simulink model "model"  (R2019a)
settings: Solver=FixedStepDiscrete  StartTime=0.0  StopTime=8  FixedStep=1/30  RelTol=1e-3  EnableMultiTasking=on
values from neighbouring files (symbols this model uses):
  A0 = 914.02    [parameter.mat]
  A1 = 12.9    [parameter.mat]
  A2 = 2028.24    [parameter.mat]
  b = 1.14    [parameter.mat]
  bpitch = 4000    [parameter.mat]
  broll = 4000    [parameter.mat]
  c = 1.14    [parameter.mat]
  C1 = 1    [parameter.mat]
  C2 = 0.34    [parameter.mat]
  C3 = 0.57    [parameter.mat]
  C4 = 0.32    [parameter.mat]
  CF = 18.7    [parameter.mat]
  f = 1.215    [parameter.mat]
  Fzt = 810    [parameter.mat]
  hs = 0.55    [parameter.mat]
  ip = 50    [parameter.mat]
  ir = 425    [parameter.mat]
  iw = 1.1    [parameter.mat]
  iz = 3136    [parameter.mat]
  Ka = 0.05    [parameter.mat]
  kpitch = 170000    [parameter.mat]
  kroll = 90000    [parameter.mat]
  m = 750    [parameter.mat]
  miudot = 0.85    [parameter.mat]
  ms = 650    [parameter.mat]
  r = 1.205    [parameter.mat]
  rw = 0.237    [parameter.mat]
  Tp = 24    [parameter.mat]
  Tw = 6    [parameter.mat]
  w = 2.28    [parameter.mat]
undefined symbols (not defined in the file or in its folder): DiscIntNeverNeededParam, Rec, SDTV, sigbuilder_block
libraries: dspmtrx3 x3, visionconversions x2, visiontextngfix x2, visiontransforms x2, fuzblock x1, dspvision x1, visionfilter x1, visionsinks x1, visionstatistics x1
(part 2 of 3)

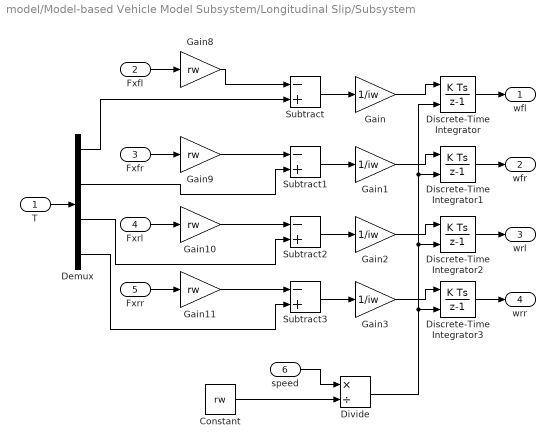
== system model/Model-based Vehicle Model Subsystem/Longitudinal Slip/Subsystem ==
  T : Inport
  Fxfl : Inport  Port=2
  Fxfr : Inport  Port=3
  Fxrl : Inport  Port=4
  Fxrr : Inport  Port=5
  speed : Inport  Port=6
  Constant : Constant  Value=rw
  Demux : Demux
  Discrete-Time Integrator{,1..3} (4 alike) : DiscreteIntegrator  InitialConditionSource=external  InitialCondition=22.222/rw  SampleTime=-1  LimitOutput=on  LowerSaturationLimit=0  ICPrevOutput=DiscIntNeverNeededParam  ICPrevScaledInput=DiscIntNeverNeededParam
  Divide : Product  Inputs=*/
  Gain{,1..3} (4 alike) : Gain  Gain=1/iw
  Gain{8..11} (4 alike) : Gain  Gain=rw
  Subtract{,1..3} (4 alike) : Sum  Inputs=-+
  wfl : Outport
  wfr : Outport  Port=2
  wrl : Outport  Port=3
  wrr : Outport  Port=4
  wires:
  Fxfl/1 -> Gain8/1
  Fxfr/1 -> Gain9/1
  Fxrl/1 -> Gain10/1
  Fxrr/1 -> Gain11/1
  Subtract/1 -> Gain/1
  Subtract1/1 -> Gain1/1
  Subtract2/1 -> Gain2/1
  Subtract3/1 -> Gain3/1
  Gain8/1 -> Subtract/1
  Gain9/1 -> Subtract1/1
  T/1 -> Demux/1
  Demux/1 -> Subtract/2
  Demux/2 -> Subtract1/2
  Demux/3 -> Subtract2/2
  Demux/4 -> Subtract3/2
  Gain/1 -> Discrete-Time Integrator/1
  Gain1/1 -> Discrete-Time Integrator1/1
  Gain2/1 -> Discrete-Time Integrator2/1
  Gain3/1 -> Discrete-Time Integrator3/1
  Discrete-Time Integrator/1 -> wfl/1
  Discrete-Time Integrator1/1 -> wfr/1
  Discrete-Time Integrator2/1 -> wrl/1
  Discrete-Time Integrator3/1 -> wrr/1
  Gain10/1 -> Subtract2/1
  Gain11/1 -> Subtract3/1
  speed/1 -> Divide/1
  Constant/1 -> Divide/2
  Divide/1 -> Discrete-Time Integrator2/2, Discrete-Time Integrator1/2, Discrete-Time Integrator/2, Discrete-Time Integrator3/2

== system model/Model-based Vehicle Model Subsystem/Longitudinal Slip/fl ==
  ax : Inport
  ay : Inport  Port=2
  Alpha_fl : Inport  Port=3
  yaw_rate : Inport  Port=4
  wfl : Inport  Port=5
  speed : Inport  Port=6
  Add1 : Sum
  Discrete-Time Integrator : DiscreteIntegrator  InitialConditionSource=external  InitialCondition=22.222  SampleTime=-1  LimitOutput=on  LowerSaturationLimit=0  ICPrevOutput=DiscIntNeverNeededParam  ICPrevScaledInput=DiscIntNeverNeededParam
  Discrete-Time Integrator1 : DiscreteIntegrator  SampleTime=-1  ICPrevOutput=DiscIntNeverNeededParam  ICPrevScaledInput=DiscIntNeverNeededParam
  Divide : Product  Inputs=*/
  Gain1 : Gain  Gain=b
  Gain2 : Gain  Gain=rw
  Math Function : Math  Operator=square  SaturateOnIntegerOverflow=on
  Math Function1 : Math  Operator=square  SaturateOnIntegerOverflow=on
  Math Function2 : Math  Operator=sqrt  SaturateOnIntegerOverflow=on
  Product1 : Product  RndMeth=Zero
  Saturation : Saturate  UpperLimit=1  LowerLimit=-1
  Subtract : Sum
  Subtract1 : Sum  Inputs=+-
  Trigonometric Function : Trigonometry  Operator=cos
  Sfl : Outport
  wires:
  ax/1 -> Discrete-Time Integrator/1
  wfl/1 -> Gain2/1
  ay/1 -> Discrete-Time Integrator1/1
  Math Function/1 -> Add1/1
  Add1/1 -> Math Function2/1
  Math Function2/1 -> Product1/1
  yaw_rate/1 -> Gain1/1
  Gain1/1 -> Subtract/2
  Subtract/1 -> Math Function1/1
  Math Function1/1 -> Add1/2
  Alpha_fl/1 -> Trigonometric Function/1
  Trigonometric Function/1 -> Product1/2
  Divide/1 -> Saturation/1
  Subtract1/1 -> Divide/1
  Product1/1 -> Divide/2, Subtract1/2
  Saturation/1 -> Sfl/1
  Gain2/1 -> Subtract1/1
  Discrete-Time Integrator/1 -> Math Function/1
  Discrete-Time Integrator1/1 -> Subtract/1
  speed/1 -> Discrete-Time Integrator/2

== system model/Model-based Vehicle Model Subsystem/Longitudinal Slip/fr ==
  ax : Inport
  vy : Inport  Port=2
  Alpha_fr : Inport  Port=3
  yaw_rate : Inport  Port=4
  wfr : Inport  Port=5
  speed : Inport  Port=6
  Add1 : Sum
  Discrete-Time Integrator : DiscreteIntegrator  InitialConditionSource=external  InitialCondition=22.222  SampleTime=-1  LimitOutput=on  LowerSaturationLimit=0  ICPrevOutput=DiscIntNeverNeededParam  ICPrevScaledInput=DiscIntNeverNeededParam
  Discrete-Time Integrator1 : DiscreteIntegrator  SampleTime=-1  ICPrevOutput=DiscIntNeverNeededParam  ICPrevScaledInput=DiscIntNeverNeededParam
  Divide : Product  Inputs=*/
  Gain1 : Gain  Gain=b
  Gain2 : Gain  Gain=rw
  Math Function : Math  Operator=square  SaturateOnIntegerOverflow=on
  Math Function1 : Math  Operator=square  SaturateOnIntegerOverflow=on
  Math Function2 : Math  Operator=sqrt  SaturateOnIntegerOverflow=on
  Product1 : Product  RndMeth=Zero
  Saturation : Saturate  UpperLimit=1  LowerLimit=-1
  Subtract : Sum
  Subtract1 : Sum  Inputs=+-
  Trigonometric Function : Trigonometry  Operator=cos
  Sfr : Outport
  wires:
  wfr/1 -> Gain2/1
  vy/1 -> Discrete-Time Integrator1/1
  Math Function/1 -> Add1/1
  Add1/1 -> Math Function2/1
  Math Function2/1 -> Product1/1
  yaw_rate/1 -> Gain1/1
  Gain1/1 -> Subtract/2
  Subtract/1 -> Math Function1/1
  Math Function1/1 -> Add1/2
  Alpha_fr/1 -> Trigonometric Function/1
  Trigonometric Function/1 -> Product1/2
  ax/1 -> Discrete-Time Integrator/1
  Subtract1/1 -> Divide/1
  Divide/1 -> Saturation/1
  Product1/1 -> Divide/2, Subtract1/2
  Saturation/1 -> Sfr/1
  Gain2/1 -> Subtract1/1
  Discrete-Time Integrator/1 -> Math Function/1
  Discrete-Time Integrator1/1 -> Subtract/1
  speed/1 -> Discrete-Time Integrator/2

== system model/Model-based Vehicle Model Subsystem/Longitudinal Slip/rl ==
  vx : Inport
  vy : Inport  Port=2
  Alpha_rl : Inport  Port=3
  yaw_rate : Inport  Port=4
  wrl : Inport  Port=5
  speed : Inport  Port=6
  Add1 : Sum
  Discrete-Time Integrator : DiscreteIntegrator  InitialConditionSource=external  InitialCondition=22.222  SampleTime=-1  LimitOutput=on  LowerSaturationLimit=0  ICPrevOutput=DiscIntNeverNeededParam  ICPrevScaledInput=DiscIntNeverNeededParam
  Discrete-Time Integrator1 : DiscreteIntegrator  SampleTime=-1  ICPrevOutput=DiscIntNeverNeededParam  ICPrevScaledInput=DiscIntNeverNeededParam
  Divide : Product  Inputs=*/
  Gain1 : Gain  Gain=c
  Gain2 : Gain  Gain=rw
  Math Function : Math  Operator=square  SaturateOnIntegerOverflow=on
  Math Function1 : Math  Operator=square  SaturateOnIntegerOverflow=on
  Math Function2 : Math  Operator=sqrt  SaturateOnIntegerOverflow=on
  Product1 : Product  RndMeth=Zero
  Saturation : Saturate  UpperLimit=1  LowerLimit=-1
  Subtract : Sum
  Subtract1 : Sum  Inputs=+-
  Trigonometric Function : Trigonometry  Operator=cos
  Srl : Outport
  wires:
  wrl/1 -> Gain2/1
  vy/1 -> Discrete-Time Integrator1/1
  Math Function/1 -> Add1/1
  Add1/1 -> Math Function2/1
  Math Function2/1 -> Product1/1
  yaw_rate/1 -> Gain1/1
  Gain1/1 -> Subtract/2
  Subtract/1 -> Math Function1/1
  Math Function1/1 -> Add1/2
  Alpha_rl/1 -> Trigonometric Function/1
  Trigonometric Function/1 -> Product1/2
  vx/1 -> Discrete-Time Integrator/1
  Subtract1/1 -> Divide/1
  Divide/1 -> Saturation/1
  Product1/1 -> Divide/2, Subtract1/2
  Saturation/1 -> Srl/1
  Gain2/1 -> Subtract1/1
  Discrete-Time Integrator/1 -> Math Function/1
  Discrete-Time Integrator1/1 -> Subtract/1
  speed/1 -> Discrete-Time Integrator/2

== system model/Model-based Vehicle Model Subsystem/Longitudinal Slip/rr ==
  vx : Inport
  vy : Inport  Port=2
  Alpha_rr : Inport  Port=3
  yaw_rate : Inport  Port=4
  wrr : Inport  Port=5
  speed : Inport  Port=6
  Add1 : Sum
  Discrete-Time Integrator : DiscreteIntegrator  InitialConditionSource=external  InitialCondition=22.222  SampleTime=-1  LimitOutput=on  LowerSaturationLimit=0  ICPrevOutput=DiscIntNeverNeededParam  ICPrevScaledInput=DiscIntNeverNeededParam
  Discrete-Time Integrator1 : DiscreteIntegrator  SampleTime=-1  ICPrevOutput=DiscIntNeverNeededParam  ICPrevScaledInput=DiscIntNeverNeededParam
  Divide : Product  Inputs=*/
  Gain1 : Gain  Gain=c
  Gain2 : Gain  Gain=rw
  Math Function : Math  Operator=square  SaturateOnIntegerOverflow=on
  Math Function1 : Math  Operator=square  SaturateOnIntegerOverflow=on
  Math Function2 : Math  Operator=sqrt  SaturateOnIntegerOverflow=on
  Product1 : Product  RndMeth=Zero
  Saturation : Saturate  UpperLimit=1  LowerLimit=-1
  Subtract : Sum
  Subtract1 : Sum  Inputs=+-
  Trigonometric Function : Trigonometry  Operator=cos
  Srr : Outport
  wires:
  wrr/1 -> Gain2/1
  vy/1 -> Discrete-Time Integrator1/1
  Math Function/1 -> Add1/1
  Add1/1 -> Math Function2/1
  Math Function2/1 -> Product1/1
  yaw_rate/1 -> Gain1/1
  Gain1/1 -> Subtract/2
  Subtract/1 -> Math Function1/1
  Math Function1/1 -> Add1/2
  Alpha_rr/1 -> Trigonometric Function/1
  Trigonometric Function/1 -> Product1/2
  vx/1 -> Discrete-Time Integrator/1
  Subtract1/1 -> Divide/1
  Divide/1 -> Saturation/1
  Product1/1 -> Divide/2, Subtract1/2
  Saturation/1 -> Srr/1
  Gain2/1 -> Subtract1/1
  Discrete-Time Integrator/1 -> Math Function/1
  Discrete-Time Integrator1/1 -> Subtract/1
  speed/1 -> Discrete-Time Integrator/2

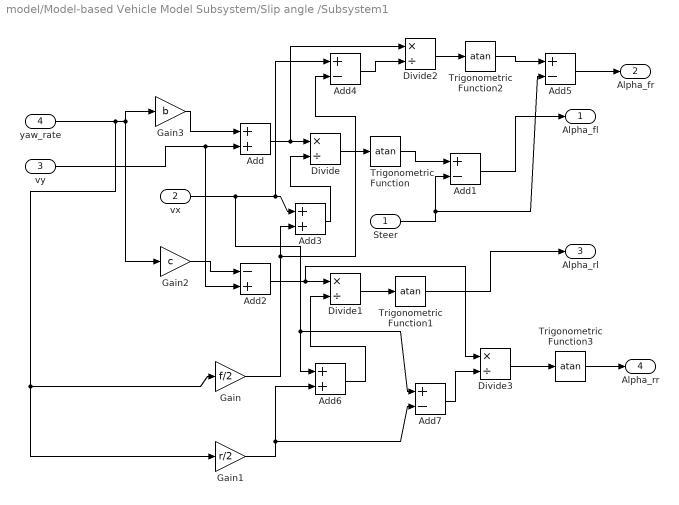
== system model/Model-based Vehicle Model Subsystem/Slip angle /Subsystem1 ==
  Steer : Inport
  vx : Inport  Port=2
  vy : Inport  Port=3
  yaw_rate : Inport  Port=4
  Add : Sum
  Add{1,4..5,7} (4 alike) : Sum  Inputs=+-
  Add2 : Sum  Inputs=-+
  Add3 : Sum
  Add6 : Sum
  Divide{,1..3} (4 alike) : Product  Inputs=*/
  Gain : Gain  Gain=f/2
  Gain1 : Gain  Gain=r/2
  Gain2 : Gain  Gain=c
  Gain3 : Gain  Gain=b
  Trigonometric Function{,1..3} (4 alike) : Trigonometry  Operator=atan
  Alpha_fl : Outport
  Alpha_fr : Outport  Port=2
  Alpha_rl : Outport  Port=3
  Alpha_rr : Outport  Port=4
  wires:
  yaw_rate/1 -> Gain1/1, Gain/1, Gain3/1, Gain2/1
  Gain3/1 -> Add/1
  vy/1 -> Add/2, Add2/2
  Add/1 -> Divide/1, Divide2/1
  Divide/1 -> Trigonometric Function/1
  Trigonometric Function/1 -> Add1/1
  Steer/1 -> Add1/2, Add5/2
  Add1/1 -> Alpha_fl/1
  Gain2/1 -> Add2/1
  Add2/1 -> Divide1/1, Divide3/1
  Divide1/1 -> Trigonometric Function1/1
  Trigonometric Function1/1 -> Alpha_rl/1
  vx/1 -> Add3/1, Add4/1, Add6/1, Add7/1
  Gain/1 -> Add3/2, Add4/2
  Add3/1 -> Divide/2
  Add4/1 -> Divide2/2
  Divide2/1 -> Trigonometric Function2/1
  Trigonometric Function2/1 -> Add5/1
  Add5/1 -> Alpha_fr/1
  Gain1/1 -> Add6/2, Add7/2
  Add6/1 -> Divide1/2
  Add7/1 -> Divide3/2
  Divide3/1 -> Trigonometric Function3/1
  Trigonometric Function3/1 -> Alpha_rr/1

== system model/Model-based Vehicle Model Subsystem/Slip angle /yaw effect motion ==
  ax : Inport
  ay : Inport  Port=2
  yaw_rate : Inport  Port=3
  speed : Inport  Port=4
  Add : Sum  Inputs=-+
  Add1 : Sum
  Discrete-Time Integrator : DiscreteIntegrator  SampleTime=-1  ICPrevOutput=DiscIntNeverNeededParam  ICPrevScaledInput=DiscIntNeverNeededParam
  Discrete-Time Integrator1 : DiscreteIntegrator  InitialConditionSource=external  InitialCondition=22.222  SampleTime=-1  LimitOutput=on  LowerSaturationLimit=0  ICPrevOutput=DiscIntNeverNeededParam  ICPrevScaledInput=DiscIntNeverNeededParam
  Product : Product  RndMeth=Zero
  Product1 : Product  RndMeth=Zero
  vx : Outport
  vy : Outport  Port=2
  wires:
  ay/1 -> Add/2
  Product/1 -> Add/1
  yaw_rate/1 -> Product/1, Product1/1
  Add/1 -> Discrete-Time Integrator/1
  Discrete-Time Integrator/1 -> vy/1, Product1/2
  ax/1 -> Add1/2
  Product1/1 -> Add1/1
  Add1/1 -> Discrete-Time Integrator1/1
  Discrete-Time Integrator1/1 -> vx/1, Product/2
  speed/1 -> Discrete-Time Integrator1/2

== system model/Model-based Vehicle Model Subsystem/Tire Model/Subsystem ==
  sfl : Inport
  Fzfl : Inport  Port=2
  Alpha_fl : Inport  Port=3
  Subsystem : Subsystem
  Subsystem1 : Subsystem
  Subsystem2 : Subsystem
  Subsystem3 : Subsystem
  Subsystem4 : Subsystem
  Subsystem5 : Subsystem
  Subsystem6 : Subsystem
  Subsystem7 : Subsystem
  Subsystem8 : Subsystem
  Unit Delay : UnitDelay  SampleTime=1/30  HasFrameUpgradeWarning=on
  Fxfl : Outport
  Fyfl : Outport  Port=2
  wires:
  Fzfl/1 -> Subsystem1/3(Fz), Subsystem2/1(Fz), Subsystem3/1(Fz), Subsystem/1(Fz), Subsystem4/2(Fz), Subsystem7/2(Fz)
  Subsystem/1(apdot) -> Subsystem1/1(apdot), Subsystem2/2(apdot), Subsystem3/2(apdot)
  Subsystem1/1(ap) -> Subsystem4/1(ap)
  Subsystem2/1(Kc) -> Subsystem4/4(Kc), Subsystem6/1(Kc)
  Subsystem3/1(Ks) -> Subsystem4/3(Ks), Subsystem6/2(Ks), Subsystem7/4(Ks), Subsystem8/3(Ks)
  sfl/1 -> Subsystem4/5(s), Subsystem6/3(s), Subsystem7/3(s)
  Alpha_fl/1 -> Subsystem4/6(Alpha), Subsystem6/4(Alpha), Subsystem7/6(Alpha), Subsystem8/5(Alpha)
  Subsystem4/1(gama) -> Subsystem5/1(gama)
  Subsystem7/1(Fx) -> Unit Delay/1, Fxfl/1
  Subsystem5/1(f(gama)) -> Subsystem7/5(f(gama)), Subsystem8/4(f(gama))
  Subsystem6/1(K'c) -> Subsystem7/1(K'c)
  Subsystem8/1(Fy) -> Fyfl/1
  Unit Delay/1 -> Subsystem1/2(Fx)
  Subsystem7/2(out1) -> Subsystem8/1(in1)
  Subsystem7/3(out2) -> Subsystem8/2(in2)

== system model/Model-based Vehicle Model Subsystem/Tire Model/Subsystem1 ==
  sfr : Inport
  Fzfr : Inport  Port=2
  Alpha_fr : Inport  Port=3
  Subsystem : Subsystem
  Subsystem1 : Subsystem
  Subsystem2 : Subsystem
  Subsystem3 : Subsystem
  Subsystem4 : Subsystem
  Subsystem5 : Subsystem
  Subsystem6 : Subsystem
  Subsystem7 : Subsystem
  Subsystem8 : Subsystem
  Unit Delay : UnitDelay  SampleTime=1/30  HasFrameUpgradeWarning=on
  Fxfr : Outport
  Fyfr : Outport  Port=2
  wires:
  Fzfr/1 -> Subsystem1/3(Fz), Subsystem2/1(Fz), Subsystem3/1(Fz), Subsystem/1(Fz), Subsystem4/2(Fz), Subsystem7/2(Fz)
  Subsystem/1(apdot) -> Subsystem1/1(apdot), Subsystem2/2(apdot), Subsystem3/2(apdot)
  Subsystem1/1(ap) -> Subsystem4/1(ap)
  Subsystem2/1(Kc) -> Subsystem4/4(Kc), Subsystem6/1(Kc)
  Subsystem3/1(Ks) -> Subsystem4/3(Ks), Subsystem6/2(Ks), Subsystem7/4(Ks), Subsystem8/3(Ks)
  sfr/1 -> Subsystem4/5(s), Subsystem6/3(s), Subsystem7/3(s)
  Alpha_fr/1 -> Subsystem4/6(Alpha), Subsystem6/4(Alpha), Subsystem7/6(Alpha), Subsystem8/5(Alpha)
  Subsystem4/1(gama) -> Subsystem5/1(gama)
  Subsystem7/1(Fx) -> Unit Delay/1, Fxfr/1
  Subsystem5/1(f(gama)) -> Subsystem7/5(f(gama)), Subsystem8/4(f(gama))
  Subsystem6/1(K'c) -> Subsystem7/1(K'c)
  Subsystem8/1(Fy) -> Fyfr/1
  Unit Delay/1 -> Subsystem1/2(Fx)
  Subsystem7/2(out1) -> Subsystem8/1(in1)
  Subsystem7/3(out2) -> Subsystem8/2(in2)

== system model/Model-based Vehicle Model Subsystem/Tire Model/Subsystem2 ==
  srl : Inport
  Fzrl : Inport  Port=2
  Alpha_rl : Inport  Port=3
  Subsystem : Subsystem
  Subsystem1 : Subsystem
  Subsystem2 : Subsystem
  Subsystem3 : Subsystem
  Subsystem4 : Subsystem
  Subsystem5 : Subsystem
  Subsystem6 : Subsystem
  Subsystem7 : Subsystem
  Subsystem8 : Subsystem
  Unit Delay : UnitDelay  SampleTime=1/30  HasFrameUpgradeWarning=on
  Fxrl : Outport
  Fyrl : Outport  Port=2
  wires:
  Fzrl/1 -> Subsystem1/3(Fz), Subsystem2/1(Fz), Subsystem3/1(Fz), Subsystem/1(Fz), Subsystem4/2(Fz), Subsystem7/2(Fz)
  Subsystem/1(apdot) -> Subsystem1/1(apdot), Subsystem2/2(apdot), Subsystem3/2(apdot)
  Subsystem1/1(ap) -> Subsystem4/1(ap)
  Subsystem2/1(Kc) -> Subsystem4/4(Kc), Subsystem6/1(Kc)
  Subsystem3/1(Ks) -> Subsystem4/3(Ks), Subsystem6/2(Ks), Subsystem7/4(Ks), Subsystem8/3(Ks)
  srl/1 -> Subsystem4/5(s), Subsystem6/3(s), Subsystem7/3(s)
  Alpha_rl/1 -> Subsystem4/6(Alpha), Subsystem6/4(Alpha), Subsystem7/6(Alpha), Subsystem8/5(Alpha)
  Subsystem4/1(gama) -> Subsystem5/1(gama)
  Subsystem7/1(Fx) -> Fxrl/1, Unit Delay/1
  Subsystem5/1(f(gama)) -> Subsystem7/5(f(gama)), Subsystem8/4(f(gama))
  Subsystem6/1(K'c) -> Subsystem7/1(K'c)
  Subsystem8/1(Fy) -> Fyrl/1
  Unit Delay/1 -> Subsystem1/2(Fx)
  Subsystem7/2(out1) -> Subsystem8/1(in1)
  Subsystem7/3(out2) -> Subsystem8/2(in2)

== system model/Model-based Vehicle Model Subsystem/Tire Model/Subsystem3 ==
  srr : Inport
  Fzrr : Inport  Port=2
  Alpha_rr : Inport  Port=3
  Subsystem : Subsystem
  Subsystem1 : Subsystem
  Subsystem2 : Subsystem
  Subsystem3 : Subsystem
  Subsystem4 : Subsystem
  Subsystem5 : Subsystem
  Subsystem6 : Subsystem
  Subsystem7 : Subsystem
  Subsystem8 : Subsystem
  Unit Delay : UnitDelay  SampleTime=1/30  HasFrameUpgradeWarning=on
  Fxrr : Outport
  Fyrr : Outport  Port=2
  wires:
  Fzrr/1 -> Subsystem1/3(Fz), Subsystem2/1(Fz), Subsystem3/1(Fz), Subsystem/1(Fz), Subsystem4/2(Fz), Subsystem7/2(Fz)
  Subsystem/1(apdot) -> Subsystem1/1(apdot), Subsystem2/2(apdot), Subsystem3/2(apdot)
  Subsystem1/1(ap) -> Subsystem4/1(ap)
  Subsystem2/1(Kc) -> Subsystem4/4(Kc), Subsystem6/1(Kc)
  Subsystem3/1(Ks) -> Subsystem4/3(Ks), Subsystem6/2(Ks), Subsystem7/4(Ks), Subsystem8/3(Ks)
  srr/1 -> Subsystem4/5(s), Subsystem6/3(s), Subsystem7/3(s)
  Alpha_rr/1 -> Subsystem4/6(Alpha), Subsystem6/4(Alpha), Subsystem7/6(Alpha), Subsystem8/5(Alpha)
  Subsystem4/1(gama) -> Subsystem5/1(gama)
  Subsystem7/1(Fx) -> Fxrr/1, Unit Delay/1
  Subsystem5/1(f(gama)) -> Subsystem7/5(f(gama)), Subsystem8/4(f(gama))
  Subsystem6/1(K'c) -> Subsystem7/1(K'c)
  Subsystem8/1(Fy) -> Fyrr/1
  Unit Delay/1 -> Subsystem1/2(Fx)
  Subsystem7/2(out1) -> Subsystem8/1(in1)
  Subsystem7/3(out2) -> Subsystem8/2(in2)

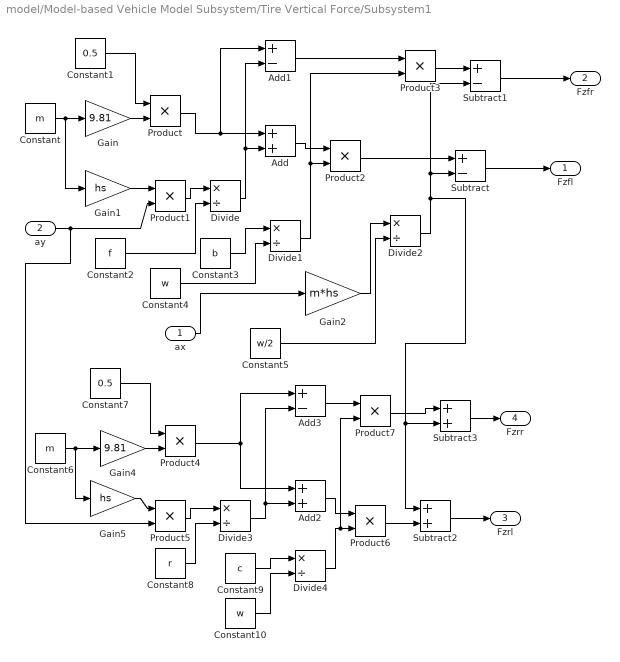
== system model/Model-based Vehicle Model Subsystem/Tire Vertical Force/Subsystem1 ==
  ax : Inport
  ay : Inport  Port=2
  Add : Sum
  Add1 : Sum  Inputs=+-
  Add2 : Sum
  Add3 : Sum  Inputs=+-
  Constant : Constant  Value=m
  Constant1 : Constant  Value=0.5
  Constant10 : Constant  Value=w
  Constant2 : Constant  Value=f
  Constant3 : Constant  Value=b
  Constant4 : Constant  Value=w
  Constant5 : Constant  Value=w/2
  Constant6 : Constant  Value=m
  Constant7 : Constant  Value=0.5
  Constant8 : Constant  Value=r
  Constant9 : Constant  Value=c
  Divide{,1..4} (5 alike) : Product  Inputs=*/
  Gain : Gain  Gain=9.81
  Gain1 : Gain  Gain=hs
  Gain2 : Gain  Gain=m*hs
  Gain4 : Gain  Gain=9.81
  Gain5 : Gain  Gain=hs
  Product{,1..7} (8 alike) : Product  RndMeth=Zero
  Subtract : Sum  Inputs=+-
  Subtract1 : Sum  Inputs=+-
  Subtract2 : Sum
  Subtract3 : Sum
  Fzfl : Outport
  Fzfr : Outport  Port=2
  Fzrl : Outport  Port=3
  Fzrr : Outport  Port=4
  wires:
  Gain/1 -> Product/2
  Constant/1 -> Gain/1, Gain1/1
  Constant1/1 -> Product/1
  Product/1 -> Add/1, Add1/1
  Gain1/1 -> Product1/1
  ay/1 -> Product1/2, Product5/2
  Product1/1 -> Divide/1
  Constant2/1 -> Divide/2
  Divide/1 -> Add/2, Add1/2
  Add/1 -> Product2/1
  Divide1/1 -> Product2/2, Product3/2
  Constant3/1 -> Divide1/1
  Constant4/1 -> Divide1/2
  Product2/1 -> Subtract/1
  ax/1 -> Gain2/1
  Gain2/1 -> Divide2/1
  Constant5/1 -> Divide2/2
  Divide2/1 -> Subtract/2, Subtract1/2, Subtract2/1, Subtract3/2
  Subtract/1 -> Fzfl/1
  Add1/1 -> Product3/1
  Product3/1 -> Subtract1/1
  Gain4/1 -> Product4/2
  Constant6/1 -> Gain4/1, Gain5/1
  Constant7/1 -> Product4/1
  Gain5/1 -> Product5/1
  Product5/1 -> Divide3/1
  Constant8/1 -> Divide3/2
  Product4/1 -> Add2/1, Add3/1
  Divide3/1 -> Add2/2, Add3/2
  Divide4/1 -> Product6/2, Product7/2
  Add2/1 -> Product6/1
  Constant9/1 -> Divide4/1
  Constant10/1 -> Divide4/2
  Product6/1 -> Subtract2/2
  Subtract1/1 -> Fzfr/1
  Subtract2/1 -> Fzrl/1
  Add3/1 -> Product7/1
  Product7/1 -> Subtract3/1
  Subtract3/1 -> Fzrr/1

== system model/Vision-based Lane Detection Subsystem/Hough Transform/Peak detection ==
  Hough : Inport
  Theta_list : Inport  Port=2
  Rho_list : Inport  Port=3
  Find Local Maxima : visionstatistics/Find Local Maxima  num_peaks=2  nhood_size=[319 89]  src_thresh=Obsolete9b  src_thresh_inuse=Specify via dialog  threshold=1  inputIsHough=on  dt_peak=uint16  isOutVarDim=on  dt_count=uint16
      settings: SourceProductName=Computer Vision Toolbox  SourceProductBaseCode=VP
  Matrix Concatenation3 : Concatenate  Mode=Multidimensional array
  Selector rho : Selector  NumberOfDimensions=2  InputPortWidth=3  IndexOptions=Select all,Index vector (port)  Indices=1,2  OutputSizes=1,1
  Selector theta : Selector  NumberOfDimensions=2  InputPortWidth=3  IndexOptions=Select all,Index vector (port)  Indices=1,2  OutputSizes=1,1
  Selector1 : Selector  NumberOfDimensions=2  InputPortWidth=3  IndexOptions=Select all,Index vector (dialog)  Indices=[2 1],[2 1]  OutputSizes=1,1
  Transpose : Math  Operator=transpose  SaturateOnIntegerOverflow=on
  Zero-Order Hold1 : ZeroOrderHold  SampleTime=-1
  Zero-Order Hold2 : ZeroOrderHold  SampleTime=-1
  select rho : Selector  NumberOfDimensions=2  InputPortWidth=3  IndexOptions=Index vector (dialog),Select all  Indices=1,-1  OutputSizes=1
  select rho3 : Selector  NumberOfDimensions=2  InputPortWidth=3  IndexOptions=Index vector (dialog),Select all  Indices=2,-1  OutputSizes=1
  Line : Outport
  wires:
  Hough/1 -> Find Local Maxima/1
  Selector theta/1 -> Matrix Concatenation3/2
  Selector rho/1 -> Matrix Concatenation3/1
  Theta_list/1 -> Zero-Order Hold1/1
  Rho_list/1 -> Zero-Order Hold2/1
  select rho/1 -> Selector rho/2
  Transpose/1 -> select rho/1, select rho3/1
  Selector1/1 -> Transpose/1
  select rho3/1 -> Selector theta/2
  Matrix Concatenation3/1 -> Line/1
  Find Local Maxima/1 -> Selector1/1
  Zero-Order Hold2/1 -> Selector rho/1
  Zero-Order Hold1/1 -> Selector theta/1

== system model/Model-based Vehicle Model Subsystem/Tire Model/Subsystem/Subsystem ==
  Fz : Inport
  Add : Sum
  Constant : Constant  Value=Fzt
  Constant1 : Constant  Value=0.0768
  Constant2 : Constant  Value=5
  Constant3 : Constant  Value=Tp
  Constant4 : Constant  Value=Tw
  Divide : Product  Inputs=*/
  Math Function : Math  Operator=sqrt  SaturateOnIntegerOverflow=on
  Product : Product  RndMeth=Zero
  Product1 : Product  RndMeth=Zero
  Product2 : Product  RndMeth=Zero
  apdot : Outport
  wires:
  Fz/1 -> Product/1
  Constant/1 -> Product/2
  Product/1 -> Math Function/1
  Math Function/1 -> Product1/1
  Constant1/1 -> Product1/2
  Product1/1 -> Divide/1
  Constant2/1 -> Add/1
  Constant3/1 -> Add/2
  Add/1 -> Product2/1
  Constant4/1 -> Product2/2
  Product2/1 -> Divide/2
  Divide/1 -> apdot/1

== system model/Model-based Vehicle Model Subsystem/Tire Model/Subsystem/Subsystem1 ==
  apdot : Inport
  Fx : Inport  Port=2
  Fz : Inport  Port=3
  Constant : Constant  Value=Ka
  Constant1 : Constant
  Divide : Product  Inputs=*/
  Product : Product  RndMeth=Zero
  Product1 : Product  RndMeth=Zero
  Subtract : Sum  Inputs=-+
  ap : Outport
  wires:
  Fx/1 -> Divide/1
  Fz/1 -> Divide/2
  Constant/1 -> Product/2
  Divide/1 -> Product/1
  Constant1/1 -> Subtract/2
  Product/1 -> Subtract/1
  apdot/1 -> Product1/1
  Subtract/1 -> Product1/2
  Product1/1 -> ap/1

== system model/Model-based Vehicle Model Subsystem/Tire Model/Subsystem/Subsystem2 ==
  Fz : Inport
  apdot : Inport  Port=2
  Constant : Constant  Value=CF
  Constant1 : Constant  Value=2
  Divide : Product  Inputs=*/
  Math Function : Math  Operator=square  SaturateOnIntegerOverflow=on
  Product : Product  RndMeth=Zero
  Product1 : Product  RndMeth=Zero
  Kc : Outport
  wires:
  Constant/1 -> Product/1
  Fz/1 -> Product/2
  apdot/1 -> Math Function/1
  Constant1/1 -> Divide/1
  Math Function/1 -> Divide/2
  Product/1 -> Product1/1
  Divide/1 -> Product1/2
  Product1/1 -> Kc/1

== system model/Model-based Vehicle Model Subsystem/Tire Model/Subsystem/Subsystem3 ==
  Fz : Inport
  apdot : Inport  Port=2
  Add : Sum
  Constant : Constant  Value=A0
  Constant1 : Constant  Value=A1
  Constant2 : Constant  Value=A1
  Constant3 : Constant  Value=A2
  Constant4 : Constant  Value=2
  Divide : Product  Inputs=*/
  Divide1 : Product  Inputs=*/
  Math Function : Math  Operator=square  SaturateOnIntegerOverflow=on
  Math Function1 : Math  Operator=square  SaturateOnIntegerOverflow=on
  Product : Product  RndMeth=Zero
  Product1 : Product  RndMeth=Zero
  Product2 : Product  RndMeth=Zero
  Terminator : Terminator
  Ks : Outport
  wires:
  Constant/1 -> Add/1
  Product/1 -> Add/2
  Constant1/1 -> Product/1
  Fz/1 -> Product/2, Math Function/1
  Constant2/1 -> Divide/1
  Constant3/1 -> Divide/2
  Divide/1 -> Product1/1
  Math Function/1 -> Product1/2
  Divide1/1 -> Product2/2
  Add/1 -> Product2/1
  Constant4/1 -> Divide1/1
  apdot/1 -> Math Function1/1
  Math Function1/1 -> Divide1/2
  Product2/1 -> Ks/1
  Product1/1 -> Terminator/1

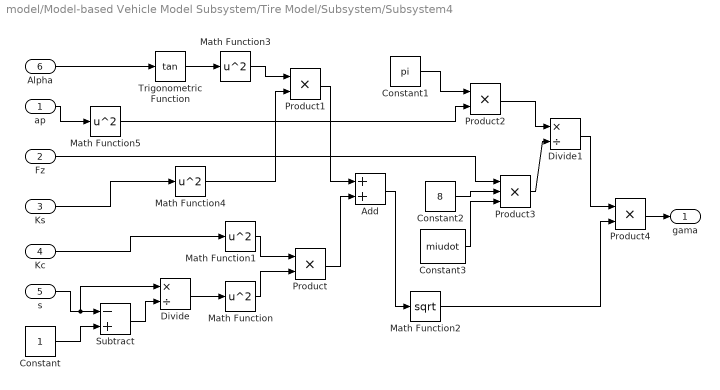
== system model/Model-based Vehicle Model Subsystem/Tire Model/Subsystem/Subsystem4 ==
  ap : Inport
  Fz : Inport  Port=2
  Ks : Inport  Port=3
  Kc : Inport  Port=4
  s : Inport  Port=5
  Alpha : Inport  Port=6
  Add : Sum
  Constant : Constant
  Constant1 : Constant  Value=pi
  Constant2 : Constant  Value=8
  Constant3 : Constant  Value=miudot
  Divide : Product  Inputs=*/
  Divide1 : Product  Inputs=*/
  Math Function{,1,3..5} (5 alike) : Math  Operator=square  SaturateOnIntegerOverflow=on
  Math Function2 : Math  Operator=sqrt  SaturateOnIntegerOverflow=on
  Product{,1..2,4} (4 alike) : Product  RndMeth=Zero
  Product3 : Product  Inputs=3  RndMeth=Zero
  Subtract : Sum  Inputs=-+
  Trigonometric Function : Trigonometry  Operator=tan
  gama : Outport
  wires:
  Constant/1 -> Subtract/2
  s/1 -> Subtract/1, Divide/1
  Subtract/1 -> Divide/2
  Divide/1 -> Math Function/1
  Kc/1 -> Math Function1/1
  Math Function1/1 -> Product/1
  Math Function/1 -> Product/2
  Product/1 -> Add/2
  Add/1 -> Math Function2/1
  Alpha/1 -> Trigonometric Function/1
  Trigonometric Function/1 -> Math Function3/1
  Math Function3/1 -> Product1/1
  Ks/1 -> Math Function4/1
  Math Function4/1 -> Product1/2
  Product1/1 -> Add/1
  Constant1/1 -> Product2/1
  ap/1 -> Math Function5/1
  Math Function5/1 -> Product2/2
  Product2/1 -> Divide1/1
  Fz/1 -> Product3/1
  Product3/1 -> Divide1/2
  Constant2/1 -> Product3/2
  Constant3/1 -> Product3/3
  Product4/1 -> gama/1
  Divide1/1 -> Product4/1
  Math Function2/1 -> Product4/2

== system model/Model-based Vehicle Model Subsystem/Tire Model/Subsystem/Subsystem5 ==
  gama : Inport
  Add : Sum  Inputs=+++
  Add1 : Sum  Inputs=++++
  Constant : Constant  Value=C1
  Constant1 : Constant  Value=C2
  Constant2 : Constant  Value=C3
  Constant3 : Constant  Value=C4
  Constant4 : Constant  Value=4
  Constant5 : Constant  Value=pi
  Constant6 : Constant
  Divide : Product  Inputs=*/
  Divide1 : Product  Inputs=*/
  Math Function : Math  Operator=square  SaturateOnIntegerOverflow=on
  Product{,1..5} (6 alike) : Product  RndMeth=Zero
  f(gama) : Outport
  wires:
  gama/1 -> Math Function/1, Product/2, Product3/1, Product5/1
  Math Function/1 -> Product/1, Product2/2, Product4/1
  Product/1 -> Product1/1
  Constant/1 -> Product1/2
  Product1/1 -> Add/1, Add1/1
  Constant1/1 -> Product2/1
  Product2/1 -> Add/2
  Constant4/1 -> Divide/1
  Constant5/1 -> Divide/2
  Divide/1 -> Product3/2
  Product3/1 -> Add/3
  Constant2/1 -> Product4/2
  Product4/1 -> Add1/2
  Product5/1 -> Add1/3
  Constant3/1 -> Product5/2
  Constant6/1 -> Add1/4
  Add/1 -> Divide1/1
  Add1/1 -> Divide1/2
  Divide1/1 -> f(gama)/1

== system model/Model-based Vehicle Model Subsystem/Tire Model/Subsystem/Subsystem6 ==
  Kc : Inport
  Ks : Inport  Port=2
  s : Inport  Port=3
  Alpha : Inport  Port=4
  Add : Sum
  Add1 : Sum
  Math Function : Math  Operator=square  SaturateOnIntegerOverflow=on
  Math Function1 : Math  Operator=square  SaturateOnIntegerOverflow=on
  Math Function2 : Math  Operator=sqrt  SaturateOnIntegerOverflow=on
  Math Function3 : Math  Operator=square  SaturateOnIntegerOverflow=on
  Product : Product  RndMeth=Zero
  Product1 : Product  RndMeth=Zero
  Subtract : Sum  Inputs=+-
  Trigonometric Function : Trigonometry  Operator=cos
  Trigonometric Function1 : Trigonometry
  K'c : Outport
  wires:
  s/1 -> Math Function/1
  Alpha/1 -> Trigonometric Function/1, Trigonometric Function1/1
  Trigonometric Function/1 -> Math Function1/1
  Math Function1/1 -> Product/2
  Math Function/1 -> Product/1
  Product/1 -> Add/2
  Add/1 -> Math Function2/1
  Trigonometric Function1/1 -> Math Function3/1
  Math Function3/1 -> Add/1
  Math Function2/1 -> Product1/2
  Ks/1 -> Subtract/1
  Kc/1 -> Subtract/2, Add1/1
  Subtract/1 -> Product1/1
  Product1/1 -> Add1/2
  Add1/1 -> K'c/1

== system model/Model-based Vehicle Model Subsystem/Tire Model/Subsystem/Subsystem7 ==
  K'c : Inport
  Fz : Inport  Port=2
  s : Inport  Port=3
  Ks : Inport  Port=4
  f(gama) : Inport  Port=5
  Alpha : Inport  Port=6
  Add : Sum
  Divide : Product  Inputs=*/
  Gain : Gain  Gain=0.85
  Math Function{,1..3} (4 alike) : Math  Operator=square  SaturateOnIntegerOverflow=on
  Math Function4 : Math  Operator=sqrt  SaturateOnIntegerOverflow=on
  Product : Product  RndMeth=Zero
  Product1 : Product  RndMeth=Zero
  Product2 : Product  Inputs=4  RndMeth=Zero
  Subsystem : Subsystem
  Trigonometric Function : Trigonometry  Operator=tan
  Fx : Outport
  out1 : Outport  Port=2
  out2 : Outport  Port=3
  wires:
  Ks/1 -> Math Function/1
  Math Function/1 -> Product/1
  Alpha/1 -> Trigonometric Function/1
  Trigonometric Function/1 -> Math Function1/1
  Math Function1/1 -> Product/2
  Product/1 -> Add/1
  K'c/1 -> Math Function2/1, Product2/4
  s/1 -> Math Function3/1, Product2/3
  Math Function2/1 -> Product1/1
  Math Function3/1 -> Product1/2
  Product1/1 -> Add/2
  Add/1 -> Math Function4/1
  Product2/1 -> Divide/1
  Fz/1 -> Gain/1
  f(gama)/1 -> Product2/2
  Divide/1 -> Fx/1
  Math Function4/1 -> Subsystem/1(In1)
  Gain/1 -> Product2/1, out2/1
  Subsystem/1(Out1) -> Divide/2, out1/1

== system model/Model-based Vehicle Model Subsystem/Tire Model/Subsystem/Subsystem8 ==
  in1 : Inport
  in2 : Inport  Port=2
  Ks : Inport  Port=3
  f(gama) : Inport  Port=4
  Alpha : Inport  Port=5
  Divide : Product  Inputs=*/
  Gain3 : Gain  Gain=-1
  Product2 : Product  Inputs=4  RndMeth=Zero
  Trigonometric Function : Trigonometry  Operator=tan
  Fy : Outport
  wires:
  Ks/1 -> Product2/4
  Alpha/1 -> Trigonometric Function/1
  Trigonometric Function/1 -> Product2/3
  Product2/1 -> Divide/1
  f(gama)/1 -> Product2/2
  Divide/1 -> Gain3/1
  in2/1 -> Product2/1
  in1/1 -> Divide/2
  Gain3/1 -> Fy/1

== system model/Model-based Vehicle Model Subsystem/Tire Model/Subsystem1/Subsystem ==
  Fz : Inport
  Add : Sum
  Constant : Constant  Value=Fzt
  Constant1 : Constant  Value=0.0768
  Constant2 : Constant  Value=5
  Constant3 : Constant  Value=Tp
  Constant4 : Constant  Value=Tw
  Divide : Product  Inputs=*/
  Math Function : Math  Operator=sqrt  SaturateOnIntegerOverflow=on
  Product : Product  RndMeth=Zero
  Product1 : Product  RndMeth=Zero
  Product2 : Product  RndMeth=Zero
  apdot : Outport
  wires:
  Fz/1 -> Product/1
  Constant/1 -> Product/2
  Product/1 -> Math Function/1
  Math Function/1 -> Product1/1
  Constant1/1 -> Product1/2
  Product1/1 -> Divide/1
  Constant2/1 -> Add/1
  Constant3/1 -> Add/2
  Add/1 -> Product2/1
  Constant4/1 -> Product2/2
  Product2/1 -> Divide/2
  Divide/1 -> apdot/1

== system model/Model-based Vehicle Model Subsystem/Tire Model/Subsystem1/Subsystem1 ==
  apdot : Inport
  Fx : Inport  Port=2
  Fz : Inport  Port=3
  Constant : Constant  Value=Ka
  Constant1 : Constant
  Divide : Product  Inputs=*/
  Product : Product  RndMeth=Zero
  Product1 : Product  RndMeth=Zero
  Subtract : Sum  Inputs=-+
  ap : Outport
  wires:
  Fx/1 -> Divide/1
  Fz/1 -> Divide/2
  Constant/1 -> Product/2
  Divide/1 -> Product/1
  Constant1/1 -> Subtract/2
  Product/1 -> Subtract/1
  apdot/1 -> Product1/1
  Subtract/1 -> Product1/2
  Product1/1 -> ap/1

== system model/Model-based Vehicle Model Subsystem/Tire Model/Subsystem1/Subsystem2 ==
  Fz : Inport
  apdot : Inport  Port=2
  Constant : Constant  Value=CF
  Constant1 : Constant  Value=2
  Divide : Product  Inputs=*/
  Math Function : Math  Operator=square  SaturateOnIntegerOverflow=on
  Product : Product  RndMeth=Zero
  Product1 : Product  RndMeth=Zero
  Kc : Outport
  wires:
  Constant/1 -> Product/1
  Fz/1 -> Product/2
  apdot/1 -> Math Function/1
  Constant1/1 -> Divide/1
  Math Function/1 -> Divide/2
  Product/1 -> Product1/1
  Divide/1 -> Product1/2
  Product1/1 -> Kc/1

== system model/Model-based Vehicle Model Subsystem/Tire Model/Subsystem1/Subsystem3 ==
  Fz : Inport
  apdot : Inport  Port=2
  Add : Sum
  Constant : Constant  Value=A0
  Constant1 : Constant  Value=A1
  Constant2 : Constant  Value=A1
  Constant3 : Constant  Value=A2
  Constant4 : Constant  Value=2
  Divide : Product  Inputs=*/
  Divide1 : Product  Inputs=*/
  Math Function : Math  Operator=square  SaturateOnIntegerOverflow=on
  Math Function1 : Math  Operator=square  SaturateOnIntegerOverflow=on
  Product : Product  RndMeth=Zero
  Product1 : Product  RndMeth=Zero
  Product2 : Product  RndMeth=Zero
  Terminator : Terminator
  Ks : Outport
  wires:
  Constant/1 -> Add/1
  Product/1 -> Add/2
  Constant1/1 -> Product/1
  Fz/1 -> Product/2, Math Function/1
  Constant2/1 -> Divide/1
  Constant3/1 -> Divide/2
  Divide/1 -> Product1/1
  Math Function/1 -> Product1/2
  Divide1/1 -> Product2/2
  Add/1 -> Product2/1
  Constant4/1 -> Divide1/1
  apdot/1 -> Math Function1/1
  Math Function1/1 -> Divide1/2
  Product2/1 -> Ks/1
  Product1/1 -> Terminator/1

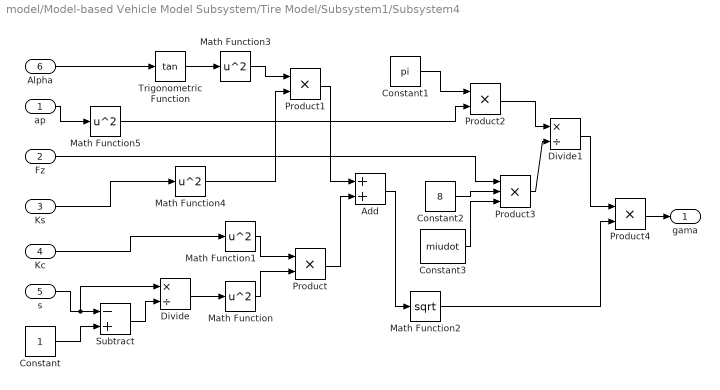
== system model/Model-based Vehicle Model Subsystem/Tire Model/Subsystem1/Subsystem4 ==
  ap : Inport
  Fz : Inport  Port=2
  Ks : Inport  Port=3
  Kc : Inport  Port=4
  s : Inport  Port=5
  Alpha : Inport  Port=6
  Add : Sum
  Constant : Constant
  Constant1 : Constant  Value=pi
  Constant2 : Constant  Value=8
  Constant3 : Constant  Value=miudot
  Divide : Product  Inputs=*/
  Divide1 : Product  Inputs=*/
  Math Function{,1,3..5} (5 alike) : Math  Operator=square  SaturateOnIntegerOverflow=on
  Math Function2 : Math  Operator=sqrt  SaturateOnIntegerOverflow=on
  Product{,1..2,4} (4 alike) : Product  RndMeth=Zero
  Product3 : Product  Inputs=3  RndMeth=Zero
  Subtract : Sum  Inputs=-+
  Trigonometric Function : Trigonometry  Operator=tan
  gama : Outport
  wires:
  Constant/1 -> Subtract/2
  s/1 -> Subtract/1, Divide/1
  Subtract/1 -> Divide/2
  Divide/1 -> Math Function/1
  Kc/1 -> Math Function1/1
  Math Function1/1 -> Product/1
  Math Function/1 -> Product/2
  Product/1 -> Add/2
  Add/1 -> Math Function2/1
  Alpha/1 -> Trigonometric Function/1
  Trigonometric Function/1 -> Math Function3/1
  Math Function3/1 -> Product1/1
  Ks/1 -> Math Function4/1
  Math Function4/1 -> Product1/2
  Product1/1 -> Add/1
  Constant1/1 -> Product2/1
  ap/1 -> Math Function5/1
  Math Function5/1 -> Product2/2
  Product2/1 -> Divide1/1
  Fz/1 -> Product3/1
  Product3/1 -> Divide1/2
  Constant2/1 -> Product3/2
  Constant3/1 -> Product3/3
  Product4/1 -> gama/1
  Divide1/1 -> Product4/1
  Math Function2/1 -> Product4/2

== system model/Model-based Vehicle Model Subsystem/Tire Model/Subsystem1/Subsystem5 ==
  gama : Inport
  Add : Sum  Inputs=+++
  Add1 : Sum  Inputs=++++
  Constant : Constant  Value=C1
  Constant1 : Constant  Value=C2
  Constant2 : Constant  Value=C3
  Constant3 : Constant  Value=C4
  Constant4 : Constant  Value=4
  Constant5 : Constant  Value=pi
  Constant6 : Constant
  Divide : Product  Inputs=*/
  Divide1 : Product  Inputs=*/
  Math Function : Math  Operator=square  SaturateOnIntegerOverflow=on
  Product{,1..5} (6 alike) : Product  RndMeth=Zero
  f(gama) : Outport
  wires:
  gama/1 -> Math Function/1, Product/2, Product3/1, Product5/1
  Math Function/1 -> Product/1, Product2/2, Product4/1
  Product/1 -> Product1/1
  Constant/1 -> Product1/2
  Product1/1 -> Add/1, Add1/1
  Constant1/1 -> Product2/1
  Product2/1 -> Add/2
  Constant4/1 -> Divide/1
  Constant5/1 -> Divide/2
  Divide/1 -> Product3/2
  Product3/1 -> Add/3
  Constant2/1 -> Product4/2
  Product4/1 -> Add1/2
  Product5/1 -> Add1/3
  Constant3/1 -> Product5/2
  Constant6/1 -> Add1/4
  Add/1 -> Divide1/1
  Add1/1 -> Divide1/2
  Divide1/1 -> f(gama)/1

== system model/Model-based Vehicle Model Subsystem/Tire Model/Subsystem1/Subsystem6 ==
  Kc : Inport
  Ks : Inport  Port=2
  s : Inport  Port=3
  Alpha : Inport  Port=4
  Add : Sum
  Add1 : Sum
  Math Function : Math  Operator=square  SaturateOnIntegerOverflow=on
  Math Function1 : Math  Operator=square  SaturateOnIntegerOverflow=on
  Math Function2 : Math  Operator=sqrt  SaturateOnIntegerOverflow=on
  Math Function3 : Math  Operator=square  SaturateOnIntegerOverflow=on
  Product : Product  RndMeth=Zero
  Product1 : Product  RndMeth=Zero
  Subtract : Sum  Inputs=+-
  Trigonometric Function : Trigonometry  Operator=cos
  Trigonometric Function1 : Trigonometry
  K'c : Outport
  wires:
  s/1 -> Math Function/1
  Alpha/1 -> Trigonometric Function/1, Trigonometric Function1/1
  Trigonometric Function/1 -> Math Function1/1
  Math Function1/1 -> Product/2
  Math Function/1 -> Product/1
  Product/1 -> Add/2
  Add/1 -> Math Function2/1
  Trigonometric Function1/1 -> Math Function3/1
  Math Function3/1 -> Add/1
  Math Function2/1 -> Product1/2
  Ks/1 -> Subtract/1
  Kc/1 -> Subtract/2, Add1/1
  Subtract/1 -> Product1/1
  Product1/1 -> Add1/2
  Add1/1 -> K'c/1

== system model/Model-based Vehicle Model Subsystem/Tire Model/Subsystem1/Subsystem7 ==
  K'c : Inport
  Fz : Inport  Port=2
  s : Inport  Port=3
  Ks : Inport  Port=4
  f(gama) : Inport  Port=5
  Alpha : Inport  Port=6
  Add : Sum
  Divide : Product  Inputs=*/
  Gain : Gain  Gain=0.85
  Math Function{,1..3} (4 alike) : Math  Operator=square  SaturateOnIntegerOverflow=on
  Math Function4 : Math  Operator=sqrt  SaturateOnIntegerOverflow=on
  Product : Product  RndMeth=Zero
  Product1 : Product  RndMeth=Zero
  Product2 : Product  Inputs=4  RndMeth=Zero
  Subsystem : Subsystem
  Trigonometric Function : Trigonometry  Operator=tan
  Fx : Outport
  out1 : Outport  Port=2
  out2 : Outport  Port=3
  wires:
  Ks/1 -> Math Function/1
  Math Function/1 -> Product/1
  Alpha/1 -> Trigonometric Function/1
  Trigonometric Function/1 -> Math Function1/1
  Math Function1/1 -> Product/2
  Product/1 -> Add/1
  K'c/1 -> Math Function2/1, Product2/4
  s/1 -> Math Function3/1, Product2/3
  Math Function2/1 -> Product1/1
  Math Function3/1 -> Product1/2
  Product1/1 -> Add/2
  Add/1 -> Math Function4/1
  Product2/1 -> Divide/1
  Fz/1 -> Gain/1
  f(gama)/1 -> Product2/2
  Divide/1 -> Fx/1
  Math Function4/1 -> Subsystem/1(In1)
  Gain/1 -> Product2/1, out2/1
  Subsystem/1(Out1) -> Divide/2, out1/1

== system model/Model-based Vehicle Model Subsystem/Tire Model/Subsystem1/Subsystem8 ==
  in1 : Inport
  in2 : Inport  Port=2
  Ks : Inport  Port=3
  f(gama) : Inport  Port=4
  Alpha : Inport  Port=5
  Divide : Product  Inputs=*/
  Gain3 : Gain  Gain=-1
  Product2 : Product  Inputs=4  RndMeth=Zero
  Trigonometric Function : Trigonometry  Operator=tan
  Fy : Outport
  wires:
  Ks/1 -> Product2/4
  Alpha/1 -> Trigonometric Function/1
  Trigonometric Function/1 -> Product2/3
  Product2/1 -> Divide/1
  f(gama)/1 -> Product2/2
  Divide/1 -> Gain3/1
  in2/1 -> Product2/1
  in1/1 -> Divide/2
  Gain3/1 -> Fy/1

== system model/Model-based Vehicle Model Subsystem/Tire Model/Subsystem2/Subsystem ==
  Fz : Inport
  Add : Sum
  Constant : Constant  Value=Fzt
  Constant1 : Constant  Value=0.0768
  Constant2 : Constant  Value=5
  Constant3 : Constant  Value=Tp
  Constant4 : Constant  Value=Tw
  Divide : Product  Inputs=*/
  Math Function : Math  Operator=sqrt  SaturateOnIntegerOverflow=on
  Product : Product  RndMeth=Zero
  Product1 : Product  RndMeth=Zero
  Product2 : Product  RndMeth=Zero
  apdot : Outport
  wires:
  Fz/1 -> Product/1
  Constant/1 -> Product/2
  Product/1 -> Math Function/1
  Math Function/1 -> Product1/1
  Constant1/1 -> Product1/2
  Product1/1 -> Divide/1
  Constant2/1 -> Add/1
  Constant3/1 -> Add/2
  Add/1 -> Product2/1
  Constant4/1 -> Product2/2
  Product2/1 -> Divide/2
  Divide/1 -> apdot/1

== system model/Model-based Vehicle Model Subsystem/Tire Model/Subsystem2/Subsystem1 ==
  apdot : Inport
  Fx : Inport  Port=2
  Fz : Inport  Port=3
  Constant : Constant  Value=Ka
  Constant1 : Constant
  Divide : Product  Inputs=*/
  Product : Product  RndMeth=Zero
  Product1 : Product  RndMeth=Zero
  Subtract : Sum  Inputs=-+
  ap : Outport
  wires:
  Fx/1 -> Divide/1
  Fz/1 -> Divide/2
  Constant/1 -> Product/2
  Divide/1 -> Product/1
  Constant1/1 -> Subtract/2
  Product/1 -> Subtract/1
  apdot/1 -> Product1/1
  Subtract/1 -> Product1/2
  Product1/1 -> ap/1

== system model/Model-based Vehicle Model Subsystem/Tire Model/Subsystem2/Subsystem2 ==
  Fz : Inport
  apdot : Inport  Port=2
  Constant : Constant  Value=CF
  Constant1 : Constant  Value=2
  Divide : Product  Inputs=*/
  Math Function : Math  Operator=square  SaturateOnIntegerOverflow=on
  Product : Product  RndMeth=Zero
  Product1 : Product  RndMeth=Zero
  Kc : Outport
  wires:
  Constant/1 -> Product/1
  Fz/1 -> Product/2
  apdot/1 -> Math Function/1
  Constant1/1 -> Divide/1
  Math Function/1 -> Divide/2
  Product/1 -> Product1/1
  Divide/1 -> Product1/2
  Product1/1 -> Kc/1

== system model/Model-based Vehicle Model Subsystem/Tire Model/Subsystem2/Subsystem3 ==
  Fz : Inport
  apdot : Inport  Port=2
  Add : Sum
  Constant : Constant  Value=A0
  Constant1 : Constant  Value=A1
  Constant2 : Constant  Value=A1
  Constant3 : Constant  Value=A2
  Constant4 : Constant  Value=2
  Divide : Product  Inputs=*/
  Divide1 : Product  Inputs=*/
  Math Function : Math  Operator=square  SaturateOnIntegerOverflow=on
  Math Function1 : Math  Operator=square  SaturateOnIntegerOverflow=on
  Product : Product  RndMeth=Zero
  Product1 : Product  RndMeth=Zero
  Product2 : Product  RndMeth=Zero
  Terminator : Terminator
  Ks : Outport
  wires:
  Constant/1 -> Add/1
  Product/1 -> Add/2
  Constant1/1 -> Product/1
  Fz/1 -> Product/2, Math Function/1
  Constant2/1 -> Divide/1
  Constant3/1 -> Divide/2
  Divide/1 -> Product1/1
  Math Function/1 -> Product1/2
  Divide1/1 -> Product2/2
  Add/1 -> Product2/1
  Constant4/1 -> Divide1/1
  apdot/1 -> Math Function1/1
  Math Function1/1 -> Divide1/2
  Product2/1 -> Ks/1
  Product1/1 -> Terminator/1

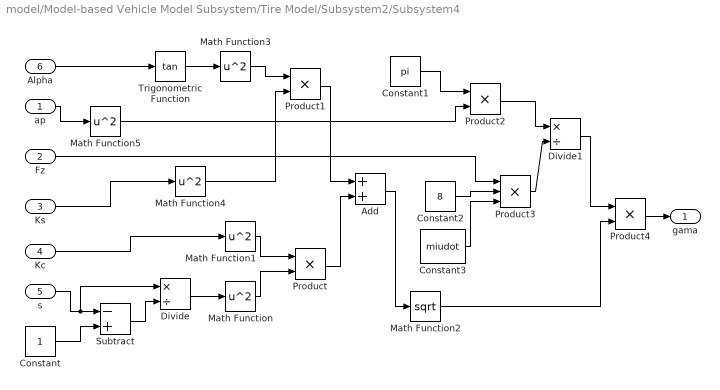
== system model/Model-based Vehicle Model Subsystem/Tire Model/Subsystem2/Subsystem4 ==
  ap : Inport
  Fz : Inport  Port=2
  Ks : Inport  Port=3
  Kc : Inport  Port=4
  s : Inport  Port=5
  Alpha : Inport  Port=6
  Add : Sum
  Constant : Constant
  Constant1 : Constant  Value=pi
  Constant2 : Constant  Value=8
  Constant3 : Constant  Value=miudot
  Divide : Product  Inputs=*/
  Divide1 : Product  Inputs=*/
  Math Function{,1,3..5} (5 alike) : Math  Operator=square  SaturateOnIntegerOverflow=on
  Math Function2 : Math  Operator=sqrt  SaturateOnIntegerOverflow=on
  Product{,1..2,4} (4 alike) : Product  RndMeth=Zero
  Product3 : Product  Inputs=3  RndMeth=Zero
  Subtract : Sum  Inputs=-+
  Trigonometric Function : Trigonometry  Operator=tan
  gama : Outport
  wires:
  Constant/1 -> Subtract/2
  s/1 -> Subtract/1, Divide/1
  Subtract/1 -> Divide/2
  Divide/1 -> Math Function/1
  Kc/1 -> Math Function1/1
  Math Function1/1 -> Product/1
  Math Function/1 -> Product/2
  Product/1 -> Add/2
  Add/1 -> Math Function2/1
  Alpha/1 -> Trigonometric Function/1
  Trigonometric Function/1 -> Math Function3/1
  Math Function3/1 -> Product1/1
  Ks/1 -> Math Function4/1
  Math Function4/1 -> Product1/2
  Product1/1 -> Add/1
  Constant1/1 -> Product2/1
  ap/1 -> Math Function5/1
  Math Function5/1 -> Product2/2
  Product2/1 -> Divide1/1
  Fz/1 -> Product3/1
  Product3/1 -> Divide1/2
  Constant2/1 -> Product3/2
  Constant3/1 -> Product3/3
  Product4/1 -> gama/1
  Divide1/1 -> Product4/1
  Math Function2/1 -> Product4/2

== system model/Model-based Vehicle Model Subsystem/Tire Model/Subsystem2/Subsystem5 ==
  gama : Inport
  Add : Sum  Inputs=+++
  Add1 : Sum  Inputs=++++
  Constant : Constant  Value=C1
  Constant1 : Constant  Value=C2
  Constant2 : Constant  Value=C3
  Constant3 : Constant  Value=C4
  Constant4 : Constant  Value=4
  Constant5 : Constant  Value=pi
  Constant6 : Constant
  Divide : Product  Inputs=*/
  Divide1 : Product  Inputs=*/
  Math Function : Math  Operator=square  SaturateOnIntegerOverflow=on
  Product{,1..5} (6 alike) : Product  RndMeth=Zero
  f(gama) : Outport
  wires:
  gama/1 -> Math Function/1, Product/2, Product3/1, Product5/1
  Math Function/1 -> Product/1, Product2/2, Product4/1
  Product/1 -> Product1/1
  Constant/1 -> Product1/2
  Product1/1 -> Add/1, Add1/1
  Constant1/1 -> Product2/1
  Product2/1 -> Add/2
  Constant4/1 -> Divide/1
  Constant5/1 -> Divide/2
  Divide/1 -> Product3/2
  Product3/1 -> Add/3
  Constant2/1 -> Product4/2
  Product4/1 -> Add1/2
  Product5/1 -> Add1/3
  Constant3/1 -> Product5/2
  Constant6/1 -> Add1/4
  Add/1 -> Divide1/1
  Add1/1 -> Divide1/2
  Divide1/1 -> f(gama)/1

== system model/Model-based Vehicle Model Subsystem/Tire Model/Subsystem2/Subsystem6 ==
  Kc : Inport
  Ks : Inport  Port=2
  s : Inport  Port=3
  Alpha : Inport  Port=4
  Add : Sum
  Add1 : Sum
  Math Function : Math  Operator=square  SaturateOnIntegerOverflow=on
  Math Function1 : Math  Operator=square  SaturateOnIntegerOverflow=on
  Math Function2 : Math  Operator=sqrt  SaturateOnIntegerOverflow=on
  Math Function3 : Math  Operator=square  SaturateOnIntegerOverflow=on
  Product : Product  RndMeth=Zero
  Product1 : Product  RndMeth=Zero
  Subtract : Sum  Inputs=+-
  Trigonometric Function : Trigonometry  Operator=cos
  Trigonometric Function1 : Trigonometry
  K'c : Outport
  wires:
  s/1 -> Math Function/1
  Alpha/1 -> Trigonometric Function/1, Trigonometric Function1/1
  Trigonometric Function/1 -> Math Function1/1
  Math Function1/1 -> Product/2
  Math Function/1 -> Product/1
  Product/1 -> Add/2
  Add/1 -> Math Function2/1
  Trigonometric Function1/1 -> Math Function3/1
  Math Function3/1 -> Add/1
  Math Function2/1 -> Product1/2
  Ks/1 -> Subtract/1
  Kc/1 -> Subtract/2, Add1/1
  Subtract/1 -> Product1/1
  Product1/1 -> Add1/2
  Add1/1 -> K'c/1

== system model/Model-based Vehicle Model Subsystem/Tire Model/Subsystem2/Subsystem7 ==
  K'c : Inport
  Fz : Inport  Port=2
  s : Inport  Port=3
  Ks : Inport  Port=4
  f(gama) : Inport  Port=5
  Alpha : Inport  Port=6
  Add : Sum
  Divide : Product  Inputs=*/
  Gain : Gain  Gain=0.85
  Math Function{,1..3} (4 alike) : Math  Operator=square  SaturateOnIntegerOverflow=on
  Math Function4 : Math  Operator=sqrt  SaturateOnIntegerOverflow=on
  Product : Product  RndMeth=Zero
  Product1 : Product  RndMeth=Zero
  Product2 : Product  Inputs=4  RndMeth=Zero
  Subsystem : Subsystem
  Trigonometric Function : Trigonometry  Operator=tan
  Fx : Outport
  out1 : Outport  Port=2
  out2 : Outport  Port=3
  wires:
  Ks/1 -> Math Function/1
  Math Function/1 -> Product/1
  Alpha/1 -> Trigonometric Function/1
  Trigonometric Function/1 -> Math Function1/1
  Math Function1/1 -> Product/2
  Product/1 -> Add/1
  K'c/1 -> Math Function2/1, Product2/4
  s/1 -> Math Function3/1, Product2/3
  Math Function2/1 -> Product1/1
  Math Function3/1 -> Product1/2
  Product1/1 -> Add/2
  Add/1 -> Math Function4/1
  Product2/1 -> Divide/1
  Fz/1 -> Gain/1
  f(gama)/1 -> Product2/2
  Divide/1 -> Fx/1
  Math Function4/1 -> Subsystem/1(In1)
  Gain/1 -> Product2/1, out2/1
  Subsystem/1(Out1) -> Divide/2, out1/1

== system model/Model-based Vehicle Model Subsystem/Tire Model/Subsystem2/Subsystem8 ==
  in1 : Inport
  in2 : Inport  Port=2
  Ks : Inport  Port=3
  f(gama) : Inport  Port=4
  Alpha : Inport  Port=5
  Divide : Product  Inputs=*/
  Gain3 : Gain  Gain=-1
  Product2 : Product  Inputs=4  RndMeth=Zero
  Trigonometric Function : Trigonometry  Operator=tan
  Fy : Outport
  wires:
  Ks/1 -> Product2/4
  Alpha/1 -> Trigonometric Function/1
  Trigonometric Function/1 -> Product2/3
  Product2/1 -> Divide/1
  f(gama)/1 -> Product2/2
  Divide/1 -> Gain3/1
  in2/1 -> Product2/1
  in1/1 -> Divide/2
  Gain3/1 -> Fy/1

== system model/Model-based Vehicle Model Subsystem/Tire Model/Subsystem3/Subsystem ==
  Fz : Inport
  Add : Sum
  Constant : Constant  Value=Fzt
  Constant1 : Constant  Value=0.0768
  Constant2 : Constant  Value=5
  Constant3 : Constant  Value=Tp
  Constant4 : Constant  Value=Tw
  Divide : Product  Inputs=*/
  Math Function : Math  Operator=sqrt  SaturateOnIntegerOverflow=on
  Product : Product  RndMeth=Zero
  Product1 : Product  RndMeth=Zero
  Product2 : Product  RndMeth=Zero
  apdot : Outport
  wires:
  Fz/1 -> Product/1
  Constant/1 -> Product/2
  Product/1 -> Math Function/1
  Math Function/1 -> Product1/1
  Constant1/1 -> Product1/2
  Product1/1 -> Divide/1
  Constant2/1 -> Add/1
  Constant3/1 -> Add/2
  Add/1 -> Product2/1
  Constant4/1 -> Product2/2
  Product2/1 -> Divide/2
  Divide/1 -> apdot/1

== system model/Model-based Vehicle Model Subsystem/Tire Model/Subsystem3/Subsystem1 ==
  apdot : Inport
  Fx : Inport  Port=2
  Fz : Inport  Port=3
  Constant : Constant  Value=Ka
  Constant1 : Constant
  Divide : Product  Inputs=*/
  Product : Product  RndMeth=Zero
  Product1 : Product  RndMeth=Zero
  Subtract : Sum  Inputs=-+
  ap : Outport
  wires:
  Fx/1 -> Divide/1
  Fz/1 -> Divide/2
  Constant/1 -> Product/2
  Divide/1 -> Product/1
  Constant1/1 -> Subtract/2
  Product/1 -> Subtract/1
  apdot/1 -> Product1/1
  Subtract/1 -> Product1/2
  Product1/1 -> ap/1
